simulink model "M10B39_V2"  (R2025a)
settings: Solver=ode23tb  StartTime=0.0  StopTime=1000  FixedStep=0.001  RelTol=1e-3  EnableMultiTasking=on
InitFcn:
  | clear;
  | initAll_V2;
  | %set_param('M10B39/Python2Sim','value','zeros(1,16)');
values from neighbouring files (symbols this model uses):
  acom = 100    [initAll.m]    (also in initAll_V2.m)
  bcom = 50    [initAll.m]    (also in initAll_V2.m)
  commun = 0*commun    [initAll.m]    (also in initAll_V2.m)
  DataDelay = 0.0*DataDelay    [initAll.m]    (also in initAll_V2.m)
  fB = 50    [initAll.m]    (also in initAll_V2.m)
  Geninit = Generator_init(opdata,SynMach_in_gidx)    [initAll.m]    (also in initAll_V2.m)
  lam = 100    [initAll.m]    (also in initAll_V2.m)
  loadnode = 31    [initAll_V2.m]
  loadsize = 16.2714    [initAll_V2.m]
  SgridB = 100    [initAll.m]    (also in initAll_V2.m)
  wB = 2*pi*fB    (= 314.159265359)    [initAll.m]    (also in initAll_V2.m)
undefined symbols (not defined in the file or in its folder): AVm0, c1, c2, c3, c4, c5, c6, cp_nom, ESinit, lambda_nom, P_wind_base, Pelec_base, Pnom, Windinit, YY_load
libraries: spsBistableLib x13, simulink_extras x5, powerlib_meascontrol x2, simulink x1
(part 3 of 11)

== system M10B39_V2/Network1 ==
  Ixy : Inport
  Assertion : Assertion  AssertionFailFcn=set_param(bdroot, 'SimulationCommand', 'pause')  StopWhenAssertionFail=off
  Clock : Clock
  Clock1 : Clock
  Constant : Constant  Value=0.001
  Mux : Mux  Inputs=2
  Relational Operator : RelationalOperator  Operator=<=  OutDataTypeStr=boolean  RndMeth=Simplest  InputSameDT=off
  Relational Operator1 : RelationalOperator  Operator=<=  OutDataTypeStr=boolean  RndMeth=Simplest  InputSameDT=off
  S-Function : S-Function  FunctionName=TS_net_1_new  Parameters=YY_load,ng,loadnode,loadsize  SFunctionDeploymentMode=off  EnableBusSupport=off
  S-Function Examples : simulink/User-Defined Functions/S-Function Examples  Commented=on
  S-Function1 : S-Function  Commented=on  Parameters=YY_load,ng  SFunctionDeploymentMode=off  EnableBusSupport=off
  Scope : Scope
      settings: ActiveDisplayYMinimum=0.9  ActiveDisplayYMaximum=1.1
  Sum : Sum  Inputs=|++
  pause_time : Constant  Value=1000
  Vxy : Outport
  wires:
  Ixy/1 -> Mux/2
  Mux/1 -> S-Function/1
  S-Function/1 -> Vxy/1
  Clock/1 -> Relational Operator/1, Mux/1
  Relational Operator/1 -> Assertion/1
  Clock1/1 -> Relational Operator1/1
  pause_time/1 -> Sum/1, Relational Operator/2
  Sum/1 -> Relational Operator1/2
  Relational Operator1/1 -> Scope/1
  Constant/1 -> Sum/2

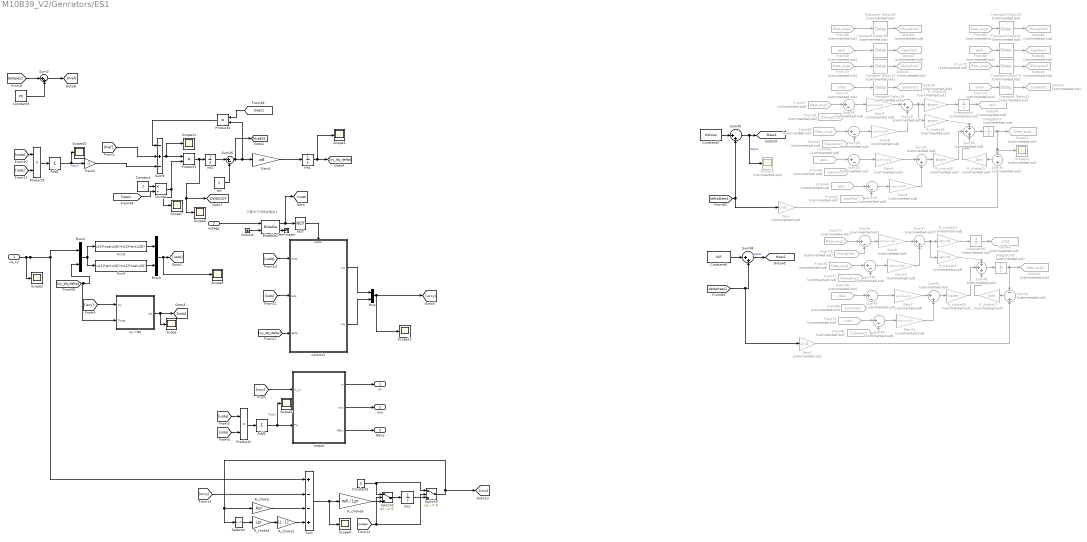
== system M10B39_V2/Genrators/ES1 ==
  note: 只要大于0就会输出1
  us_xy : Inport
  outage : Inport  Port=2
  " control1" : Subsystem
  Add1 : Sum  Inputs=+
  Add2 : Sum  Inputs=+
  Bistable2 : spsBistableLib/Bistable  Qpriority=Set  ic=0  Ts=0
      settings: LibrarySourceBlock=sps_lib/Control/Bistable
  Constant : Constant
  Constant1 : Constant  Value=0
  Constant3 : Constant  Value=P0
  Constant5 : Constant  Value=Kdroop
  Constant6 : Constant  Value=KIR
  Divide : Product  Inputs=*/
  Fcn3 : Fcn  Expr=u(1)*cos(u(3))+u(2)*sin(u(3))
  Fcn4 : Fcn  Expr=-u(1)*sin(u(3))+u(2)*cos(u(3))
  From57 : From  Commented=on  GotoTag=Dess_avg1  TagVisibility=global
  From58 : From  Commented=on  GotoTag=Dess_avg2  TagVisibility=global
  From59 : From  Commented=on  GotoTag=Dess_avg1  TagVisibility=global
  From60 : From  Commented=on  GotoTag=Dess_avg4  TagVisibility=global
  From61 : From  Commented=on  GotoTag=Davg2rec
  From62 : From  Commented=on  GotoTag=Davg4rec
  From63 : From  Commented=on  GotoTag=epi1  TagVisibility=global
  From64 : From  Commented=on  GotoTag=epi1  TagVisibility=global
  From66 : From  Commented=on  GotoTag=epi2rec
  From67 : From  Commented=on  GotoTag=epi4rec
  From68 : From  Commented=on  GotoTag=epi2  TagVisibility=global
  From69 : From  Commented=on  GotoTag=epi4  TagVisibility=global
  From70 : From  Commented=on  GotoTag=Hess_avg2  TagVisibility=global
  From71 : From  Commented=on  GotoTag=yita2  TagVisibility=global
  From72 : From  Commented=on  GotoTag=Hess_avg4  TagVisibility=global
  From73 : From  Commented=on  GotoTag=yita4  TagVisibility=global
  From74 : From  Commented=on  GotoTag=Hess_avg1  TagVisibility=global
  From75 : From  Commented=on  GotoTag=Hess_avg1  TagVisibility=global
  From76 : From  Commented=on  GotoTag=Havg2rec
  From77 : From  Commented=on  GotoTag=Havg4rec
  From78 : From  Commented=on  GotoTag=yita1  TagVisibility=global
  From79 : From  Commented=on  GotoTag=yita1  TagVisibility=global
  From80 : From  Commented=on  GotoTag=yita2rec
  From81 : From  Commented=on  GotoTag=yita4rec
  Gain : Gain  Commented=on  Gain=0.01
  Gain1 : Gain  Gain=wB  SaturateOnIntegerOverflow=on  OutDataTypeStr=Inherit: Same as input  ParamDataTypeStr=Inherit: Same as input
  Gain{8..11} (4 alike) : Gain  Commented=on  Gain=commun(4)
  Gain2 : Gain  Commented=on  Gain=0.01
  Gain{3,5..7} (4 alike) : Gain  Commented=on  Gain=commun(1)
  Gain4 : Gain  Gain=-1
  Goto32 : Goto  Commented=on  GotoTag=Dess_avg1  TagVisibility=global
  Goto33 : Goto  Commented=on  GotoTag=Havg2rec
  Goto34 : Goto  Commented=on  GotoTag=epi1  TagVisibility=global
  Goto35 : Goto  Commented=on  GotoTag=Davg2rec
  Goto36 : Goto  Commented=on  GotoTag=Davg4rec
  Goto37 : Goto  Commented=on  GotoTag=epi2rec
  Goto38 : Goto  Commented=on  GotoTag=epi4rec
  Goto39 : Goto  Commented=on  GotoTag=yita2rec
  Goto40 : Goto  Commented=on  GotoTag=Havg4rec
  Goto41 : Goto  Commented=on  GotoTag=yita4rec
  Goto42 : Goto  Commented=on  GotoTag=Hess_avg1  TagVisibility=global
  Goto43 : Goto  Commented=on  GotoTag=yita1  TagVisibility=global
  Ground : Ground
  Int1 : Integrator  InitialCondition=Dels_hvdc
  Int2 : Integrator  InitialCondition=1
  Integrator{6..9} (4 alike) : Integrator  Commented=on
  Isxy : Integrator  InitialCondition=[Is_xA_0 Is_yA_0]
  Mux : Mux  Inputs=2
  Mux3 : Mux  Inputs=2
  Mux4 : Mux  Inputs=2
  NOT : Logic  Operator=NOT  AllPortsSameDT=off  OutDataTypeStr=boolean
  Product1 : Product
  Product2 : Product  RndMeth=Zero
  Product3 : Product  RndMeth=Zero
  Product4 : Product
  R_choke : Gain  Gain=Rpr  SaturateOnIntegerOverflow=on  OutDataTypeStr=Inherit: Same as input  ParamDataTypeStr=Inherit: Same as input
  R_choke1 : Gain  Gain=Lpr  SaturateOnIntegerOverflow=on  OutDataTypeStr=Inherit: Same as input  ParamDataTypeStr=Inherit: Same as input
  R_choke14 : Gain  Commented=on  Gain=-bcom  SaturateOnIntegerOverflow=on  OutDataTypeStr=Inherit: Same as input  ParamDataTypeStr=Inherit: Same as input
  R_choke15 : Gain  Commented=on  Gain=-acom  SaturateOnIntegerOverflow=on  OutDataTypeStr=Inherit: Same as input  ParamDataTypeStr=Inherit: Same as input
  R_choke16 : Gain  Commented=on  Gain=bcom  SaturateOnIntegerOverflow=on  OutDataTypeStr=Inherit: Same as input  ParamDataTypeStr=Inherit: Same as input
  R_choke17 : Gain  Commented=on  Gain=lam  SaturateOnIntegerOverflow=on  OutDataTypeStr=Inherit: Same as input  ParamDataTypeStr=Inherit: Same as input
  R_choke18 : Gain  Commented=on  Gain=-bcom  SaturateOnIntegerOverflow=on  OutDataTypeStr=Inherit: Same as input  ParamDataTypeStr=Inherit: Same as input
  R_choke19 : Gain  Commented=on  Gain=-acom  SaturateOnIntegerOverflow=on  OutDataTypeStr=Inherit: Same as input  ParamDataTypeStr=Inherit: Same as input
  R_choke2 : Gain  Gain=[1 -1]  SaturateOnIntegerOverflow=on  OutDataTypeStr=Inherit: Same as input  ParamDataTypeStr=Inherit: Same as input
  R_choke20 : Gain  Commented=on  Gain=bcom  SaturateOnIntegerOverflow=on  OutDataTypeStr=Inherit: Same as input  ParamDataTypeStr=Inherit: Same as input
  R_choke21 : Gain  Commented=on  Gain=lam  SaturateOnIntegerOverflow=on  OutDataTypeStr=Inherit: Same as input  ParamDataTypeStr=Inherit: Same as input
  R_choke3 : Gain  Gain=wB / Lpr  SaturateOnIntegerOverflow=on  OutDataTypeStr=Inherit: Same as input  ParamDataTypeStr=Inherit: Same as input
  Scope{,1..7,10..12} (11 alike) : Scope
      Scope settings: ActiveDisplayYMinimum=-0.0194  ActiveDisplayYMaximum=0.04689
      Scope1 settings: DataLoggingVariableName=ScopeData16
      Scope10 settings: ActiveDisplayYMinimum=-5.21032  ActiveDisplayYMaximum=-1.08346
      Scope11 settings: ActiveDisplayYMinimum=-0.1125  ActiveDisplayYMaximum=0.0125  DataLoggingVariableName=ScopeData2
      Scope12 settings: ActiveDisplayYMinimum=0.46883  ActiveDisplayYMaximum=1.25548  DataLoggingVariableName=ScopeData3
      Scope2 settings: DataLoggingVariableName=ScopeData17
      Scope3 settings: ActiveDisplayYMinimum=-0.44976  ActiveDisplayYMaximum=2.17603
      Scope4 settings: ActiveDisplayYMinimum=-2.8E-5  ActiveDisplayYMaximum=2.4E-5  DataLoggingVariableName=ScopeData5
      Scope5 settings: ActiveDisplayYMinimum=-2.50000000003  ActiveDisplayYMaximum=-2.49999999989  DataLoggingVariableName=ScopeData7
      Scope6 settings: ActiveDisplayYMinimum=-0.00021  ActiveDisplayYMaximum=0.0004  DataLoggingVariableName=ScopeData4
      Scope7 settings: ActiveDisplayYMinimum=0.9  ActiveDisplayYMaximum=1.1  DataLoggingVariableName=ScopeData14
  Scope14 : Scope  Commented=on
      settings: ActiveDisplayYMinimum=-0.0418  ActiveDisplayYMaximum=0.37621  DataLoggingVariableName=ScopeData2
  Scope15 : Scope  Commented=on
      settings: ActiveDisplayYMinimum=-1  ActiveDisplayYMaximum=1  DataLoggingVariableName=ScopeData3
  Selector : Selector  InputPortWidth=2  IndexOptions=Index vector (dialog)  Indices=[2 1]  OutputSizes=1
  Sum : Sum  Inputs=+--+  SaturateOnIntegerOverflow=on
  Sum2 : Sum  Inputs=|++
  Sum26 : Sum  Inputs=|+-  SaturateOnIntegerOverflow=on
  Sum{28,30,32,34,36,39,41,43} (8 alike) : Sum  Commented=on  Inputs=|+-  SaturateOnIntegerOverflow=on
  Sum{29,33,37,42} (4 alike) : Sum  Commented=on  Inputs=|++  SaturateOnIntegerOverflow=on
  Sum31 : Sum  Commented=on  Inputs=+++  SaturateOnIntegerOverflow=on
  Sum35 : Sum  Commented=on  Inputs=-+  SaturateOnIntegerOverflow=on
  Sum38 : Sum  Inputs=|++  SaturateOnIntegerOverflow=on
  Sum40 : Sum  Commented=on  Inputs=+++  SaturateOnIntegerOverflow=on
  Sum44 : Sum  Commented=on  Inputs=-+  SaturateOnIntegerOverflow=on
  Sum45 : Sum  Inputs=|++  SaturateOnIntegerOverflow=on
  Sum9 : Sum  Inputs=-+-  SaturateOnIntegerOverflow=on
  Switch2 : Switch  Criteria=u2 ~= 0  Threshold=0.5  InputSameDT=off
  Switch3 : Switch  Criteria=u2 ~= 0  Threshold=0.5  InputSameDT=off
  Terminator : Terminator
  Transport Delay{14..15,19,21} (4 alike) : TransportDelay  Commented=on  DelayTime=DataDelay(4,2)
  Transport Delay{18,20,22..23} (4 alike) : TransportDelay  Commented=on  DelayTime=DataDelay(2,1)
  output : Subsystem
  w0 : Constant
  xy->dq : Subsystem
  m : Outport
  isxy : Outport  Port=2
  GBxy : Outport  Port=3
  tag scope: DWES1DT=global, Dess1=global, Hess1=global, WreES1=global
  wires:
  Selector/1 -> R_choke1/1
  Sum/1 -> Scope4/1, R_choke3/1
  R_choke3/1 -> Switch2/3
  Ground/1 -> Bistable2/2
  R_choke2/1 -> Sum/4
  R_choke/1 -> Sum/3
  [ucxy] -> Sum/2
  output/1(m) -> m/1
  NOT/1 -> " control1"/Enable
  R_choke1/1 -> R_choke2/1
  Bistable2/1 -> NOT/1, [outage]
  Isxy/1 -> Switch3/3
  [isxy] -> xy->dq/1(Ixy)
  [isxy] -> output/1(is_xy)
  output/2(isxy) -> isxy/1
  [xy_dq_delta] -> " control1"/3(delta)
  xy->dq/1(Idq) -> [isdq], Scope/1
  Bistable2/2 -> Terminator/1
  outage/1 -> Bistable2/1
  [outage] -> Switch2/2, Switch3/2
  [isdq] -> " control1"/2(isdq)
  " control1"/1(ucx) -> Mux/1
  Switch2/1 -> Isxy/1
  Switch3/1 -> R_choke/1, Selector/1, [isxy]
  Mux/1 -> Scope12/1, [ucxy]
  [usdq] -> " control1"/1(usdq)
  output/3(GBxy) -> GBxy/1
  Constant1/1 -> Switch2/1, Switch3/1
  " control1"/2(ucy) -> Mux/2
  [usdq] -> Product2/1
  Add1/1 -> Scope5/1, output/2(Pe)  "Pess1"
  Product2/1 -> Add1/1
  [isdq] -> Product2/2
  Product1/1 -> Scope6/1, [DWES1DT], Int2/1
  Sum26/1 -> [WreES1], Product4/2, Gain1/1
  Int2/1 -> Sum26/1
  w0/1 -> Sum26/2
  Sum9/1 -> Product1/1, Scope11/1
  Constant/1 -> Divide/1
  Divide/1 -> Product1/2, Scope7/1
  [Hess1] -> Divide/2
  us_xy/1 -> Scope2/1, Mux4/1, Sum/1
  Fcn3/1 -> Mux3/1
  Fcn4/1 -> Mux3/2
  Mux4/1 -> Fcn3/1, Fcn4/1
  [xy_dq_delta] -> Mux4/2, xy->dq/2(Theta)
  Mux3/1 -> Scope3/1, [usdq]
  Gain4/1 -> Sum9/3
  Product4/1 -> Sum9/1
  Int1/1 -> Scope1/1, [xy_dq_delta]
  Add2/1 -> Gain4/1, Scope10/1  "Pess1"
  [usdq] -> Product3/1
  [isdq] -> Product3/2
  Product3/1 -> Add2/1
  Transport Delay19/1 -> Goto36/1
  R_choke20/1 -> Sum31/2
  R_choke19/1 -> Sum31/1
  From57/1 -> Sum28/1
  From59/1 -> Sum30/1
  Sum38/1 -> [Hess1]  "Hess1"
  Sum45/1 -> Scope15/1, [Dess1]  "Dess1"
  Constant6/1 -> Sum38/1
  From64/1 -> Sum34/1
  R_choke21/1 -> Sum31/3
  Integrator6/1 -> Goto34/1
  Sum35/1 -> R_choke21/1
  Sum31/1 -> Integrator7/1
  Integrator7/1 -> Goto32/1, Scope14/1, Sum35/1
  Transport Delay21/1 -> Goto38/1
  From68/1 -> Transport Delay20/1
  From67/1 -> Sum34/2
  From62/1 -> Sum30/2
  From80/1 -> Sum41/2
  From78/1 -> Sum41/1
  Sum40/1 -> Integrator9/1
  [deltaDess1] -> Sum45/2, Gain/1
  R_choke18/1 -> Integrator6/1
  From77/1 -> Sum39/2
  From63/1 -> Sum32/1
  From76/1 -> Sum36/2
  Sum42/1 -> R_choke16/1
  From58/1 -> Transport Delay18/1
  Transport Delay20/1 -> Goto37/1
  Transport Delay14/1 -> Goto40/1
  From75/1 -> Sum39/1
  Integrator9/1 -> Goto42/1, Sum44/1
  Sum29/1 -> R_choke19/1, R_choke18/1
  From61/1 -> Sum28/2
  From71/1 -> Transport Delay23/1
  Sum37/1 -> R_choke15/1, R_choke14/1
  R_choke14/1 -> Integrator8/1
  Integrator8/1 -> Goto43/1
  Transport Delay18/1 -> Goto35/1
  R_choke17/1 -> Sum40/3
  R_choke15/1 -> Sum40/1
  R_choke16/1 -> Sum40/2
  From74/1 -> Sum36/1
  [deltaHess1] -> Sum38/2, Gain2/1
  Sum44/1 -> R_choke17/1
  Sum33/1 -> R_choke20/1
  Transport Delay23/1 -> Goto39/1
  From66/1 -> Sum32/2
  Transport Delay22/1 -> Goto33/1
  Transport Delay15/1 -> Goto41/1
  From70/1 -> Transport Delay22/1
  [Dess1] -> Product4/1
  Gain1/1 -> Int1/1
  From81/1 -> Sum43/2
  From79/1 -> Sum43/1
  Gain/1 -> Sum35/2
  Gain2/1 -> Sum44/2
  From60/1 -> Transport Delay19/1
  From69/1 -> Transport Delay21/1
  From72/1 -> Transport Delay14/1
  From73/1 -> Transport Delay15/1
  Gain3/1 -> Sum29/1
  Sum28/1 -> Gain3/1
  Gain5/1 -> Sum33/1
  Sum32/1 -> Gain5/1
  Sum36/1 -> Gain6/1
  Gain6/1 -> Sum37/1
  Gain7/1 -> Sum42/1
  Sum41/1 -> Gain7/1
  Sum30/1 -> Gain8/1
  Gain8/1 -> Sum29/2
  Sum34/1 -> Gain9/1
  Gain9/1 -> Sum33/2
  Sum39/1 -> Gain10/1
  Gain10/1 -> Sum37/2
  Sum43/1 -> Gain11/1
  Gain11/1 -> Sum42/2
  Constant5/1 -> Sum45/1
  [deltapes1] -> Sum2/1
  Constant3/1 -> Sum2/2
  Sum2/1 -> [Pref]
  [Pref] -> Sum9/2

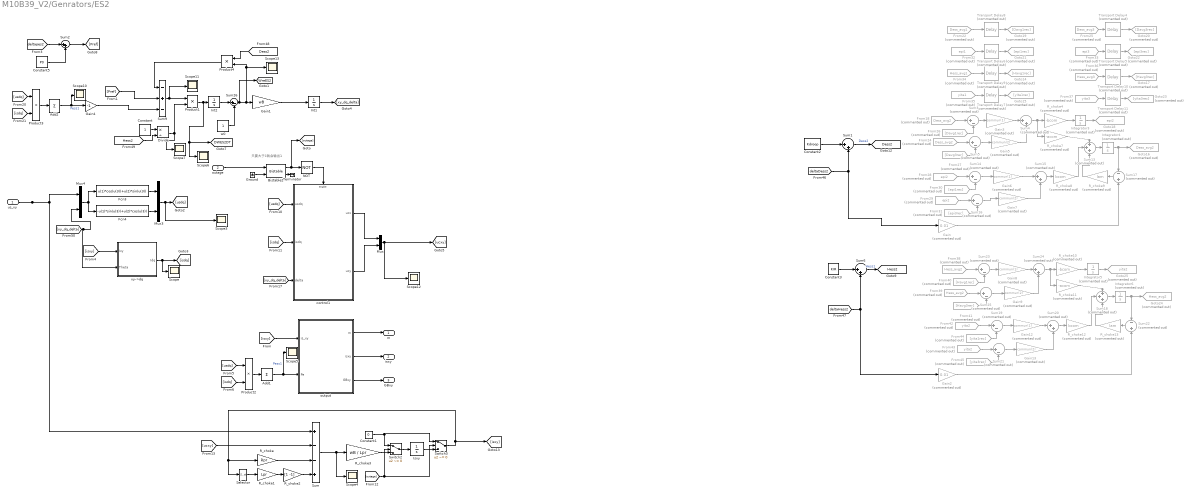
== system M10B39_V2/Genrators/ES2 ==
  note: 只要大于0就会输出1
  us_xy : Inport
  outage : Inport  Port=2
  " control1" : Subsystem
  Add1 : Sum  Inputs=+
  Add2 : Sum  Inputs=+
  Bistable2 : spsBistableLib/Bistable  Qpriority=Set  ic=0  Ts=0
      settings: LibrarySourceBlock=sps_lib/Control/Bistable
  Constant : Constant
  Constant1 : Constant  Value=0
  Constant2 : Constant  Value=Kdroop
  Constant3 : Constant  Value=KIR
  Constant5 : Constant  Value=P0
  Divide : Product  Inputs=*/
  Fcn3 : Fcn  Expr=u(1)*cos(u(3))+u(2)*sin(u(3))
  Fcn4 : Fcn  Expr=-u(1)*sin(u(3))+u(2)*cos(u(3))
  From18 : From  Commented=on  GotoTag=Dess_avg2  TagVisibility=global
  From22 : From  Commented=on  GotoTag=Dess_avg1  TagVisibility=global
  From24 : From  Commented=on  GotoTag=Dess_avg2  TagVisibility=global
  From25 : From  Commented=on  GotoTag=Dess_avg3  TagVisibility=global
  From26 : From  Commented=on  GotoTag=Davg1rec
  From27 : From  Commented=on  GotoTag=Davg3rec
  From28 : From  Commented=on  GotoTag=epi2  TagVisibility=global
  From29 : From  Commented=on  GotoTag=epi2  TagVisibility=global
  From30 : From  Commented=on  GotoTag=epi1rec
  From31 : From  Commented=on  GotoTag=epi3rec
  From32 : From  Commented=on  GotoTag=epi1  TagVisibility=global
  From33 : From  Commented=on  GotoTag=epi3  TagVisibility=global
  From34 : From  Commented=on  GotoTag=Hess_avg1  TagVisibility=global
  From35 : From  Commented=on  GotoTag=yita1  TagVisibility=global
  From36 : From  Commented=on  GotoTag=Hess_avg3  TagVisibility=global
  From37 : From  Commented=on  GotoTag=yita3  TagVisibility=global
  From38 : From  Commented=on  GotoTag=Hess_avg2  TagVisibility=global
  From39 : From  Commented=on  GotoTag=Hess_avg2  TagVisibility=global
  From40 : From  Commented=on  GotoTag=Havg1rec
  From41 : From  Commented=on  GotoTag=Havg3rec
  From42 : From  Commented=on  GotoTag=yita2  TagVisibility=global
  From43 : From  Commented=on  GotoTag=yita2  TagVisibility=global
  From44 : From  Commented=on  GotoTag=yita1rec
  From45 : From  Commented=on  GotoTag=yita3rec
  Gain : Gain  Commented=on  Gain=0.01
  Gain1 : Gain  Gain=wB  SaturateOnIntegerOverflow=on  OutDataTypeStr=Inherit: Same as input  ParamDataTypeStr=Inherit: Same as input
  Gain{3,6,8,12} (4 alike) : Gain  Commented=on  Gain=commun(1)
  Gain{5,7,9,13} (4 alike) : Gain  Commented=on  Gain=commun(2)
  Gain2 : Gain  Commented=on  Gain=0.01
  Gain4 : Gain  Gain=-1
  Goto14 : Goto  Commented=on  GotoTag=Havg1rec
  Goto15 : Goto  Commented=on  GotoTag=yita1rec
  Goto16 : Goto  Commented=on  GotoTag=Dess_avg2  TagVisibility=global
  Goto17 : Goto  Commented=on  GotoTag=Havg3rec
  Goto18 : Goto  Commented=on  GotoTag=epi2  TagVisibility=global
  Goto19 : Goto  Commented=on  GotoTag=Davg1rec
  Goto20 : Goto  Commented=on  GotoTag=Davg3rec
  Goto21 : Goto  Commented=on  GotoTag=epi1rec
  Goto22 : Goto  Commented=on  GotoTag=epi3rec
  Goto23 : Goto  Commented=on  GotoTag=yita3rec
  Goto24 : Goto  Commented=on  GotoTag=Hess_avg2  TagVisibility=global
  Goto25 : Goto  Commented=on  GotoTag=yita2  TagVisibility=global
  Ground : Ground
  Int1 : Integrator  InitialCondition=Dels_hvdc
  Int2 : Integrator  InitialCondition=1
  Integrator{3..6} (4 alike) : Integrator  Commented=on
  Isxy : Integrator  InitialCondition=[Is_xA_0 Is_yA_0]
  Mux : Mux  Inputs=2
  Mux3 : Mux  Inputs=2
  Mux4 : Mux  Inputs=2
  NOT : Logic  Operator=NOT  AllPortsSameDT=off  OutDataTypeStr=boolean
  Product1 : Product
  Product2 : Product  RndMeth=Zero
  Product3 : Product  RndMeth=Zero
  Product4 : Product
  R_choke : Gain  Gain=Rpr  SaturateOnIntegerOverflow=on  OutDataTypeStr=Inherit: Same as input  ParamDataTypeStr=Inherit: Same as input
  R_choke1 : Gain  Gain=Lpr  SaturateOnIntegerOverflow=on  OutDataTypeStr=Inherit: Same as input  ParamDataTypeStr=Inherit: Same as input
  R_choke10 : Gain  Commented=on  Gain=-bcom  SaturateOnIntegerOverflow=on  OutDataTypeStr=Inherit: Same as input  ParamDataTypeStr=Inherit: Same as input
  R_choke11 : Gain  Commented=on  Gain=-acom  SaturateOnIntegerOverflow=on  OutDataTypeStr=Inherit: Same as input  ParamDataTypeStr=Inherit: Same as input
  R_choke12 : Gain  Commented=on  Gain=bcom  SaturateOnIntegerOverflow=on  OutDataTypeStr=Inherit: Same as input  ParamDataTypeStr=Inherit: Same as input
  R_choke13 : Gain  Commented=on  Gain=lam  SaturateOnIntegerOverflow=on  OutDataTypeStr=Inherit: Same as input  ParamDataTypeStr=Inherit: Same as input
  R_choke2 : Gain  Gain=[1 -1]  SaturateOnIntegerOverflow=on  OutDataTypeStr=Inherit: Same as input  ParamDataTypeStr=Inherit: Same as input
  R_choke3 : Gain  Gain=wB / Lpr  SaturateOnIntegerOverflow=on  OutDataTypeStr=Inherit: Same as input  ParamDataTypeStr=Inherit: Same as input
  R_choke4 : Gain  Commented=on  Gain=-bcom  SaturateOnIntegerOverflow=on  OutDataTypeStr=Inherit: Same as input  ParamDataTypeStr=Inherit: Same as input
  R_choke7 : Gain  Commented=on  Gain=-acom  SaturateOnIntegerOverflow=on  OutDataTypeStr=Inherit: Same as input  ParamDataTypeStr=Inherit: Same as input
  R_choke8 : Gain  Commented=on  Gain=bcom  SaturateOnIntegerOverflow=on  OutDataTypeStr=Inherit: Same as input  ParamDataTypeStr=Inherit: Same as input
  R_choke9 : Gain  Commented=on  Gain=lam  SaturateOnIntegerOverflow=on  OutDataTypeStr=Inherit: Same as input  ParamDataTypeStr=Inherit: Same as input
  Scope{,3..7,10..13} (10 alike) : Scope
      Scope settings: ActiveDisplayYMinimum=-0.0194  ActiveDisplayYMaximum=0.04689
      Scope10 settings: ActiveDisplayYMinimum=-0.00511  ActiveDisplayYMaximum=0.046
      Scope11 settings: ActiveDisplayYMinimum=-0.1125  ActiveDisplayYMaximum=0.0125  DataLoggingVariableName=ScopeData2
      Scope12 settings: ActiveDisplayYMinimum=0.46883  ActiveDisplayYMaximum=1.25548  DataLoggingVariableName=ScopeData3
      Scope13 settings: ActiveDisplayYMinimum=-0.0063  ActiveDisplayYMaximum=0.05669  DataLoggingVariableName=ScopeData4
      Scope3 settings: ActiveDisplayYMinimum=-0.12696  ActiveDisplayYMaximum=1.14248
      Scope4 settings: ActiveDisplayYMinimum=-2.8E-5  ActiveDisplayYMaximum=2.4E-5  DataLoggingVariableName=ScopeData5
      Scope5 settings: ActiveDisplayYMinimum=-0.00823  ActiveDisplayYMaximum=0.07404  DataLoggingVariableName=ScopeData7
      Scope6 settings: ActiveDisplayYMinimum=-0.00105  ActiveDisplayYMaximum=0.00091  DataLoggingVariableName=ScopeData4
      Scope7 settings: ActiveDisplayYMinimum=0.9  ActiveDisplayYMaximum=1.1  DataLoggingVariableName=ScopeData14
  Selector : Selector  InputPortWidth=2  IndexOptions=Index vector (dialog)  Indices=[2 1]  OutputSizes=1
  Sum : Sum  Inputs=+--+  SaturateOnIntegerOverflow=on
  Sum1 : Sum  Inputs=|++  SaturateOnIntegerOverflow=on
  Sum13 : Sum  Commented=on  Inputs=+++  SaturateOnIntegerOverflow=on
  Sum{3,5,14,16,19,21,23,25} (8 alike) : Sum  Commented=on  Inputs=|+-  SaturateOnIntegerOverflow=on
  Sum{4,15,20,24} (4 alike) : Sum  Commented=on  Inputs=|++  SaturateOnIntegerOverflow=on
  Sum17 : Sum  Commented=on  Inputs=-+  SaturateOnIntegerOverflow=on
  Sum18 : Sum  Commented=on  Inputs=+++  SaturateOnIntegerOverflow=on
  Sum2 : Sum  Inputs=|++
  Sum22 : Sum  Commented=on  Inputs=-+  SaturateOnIntegerOverflow=on
  Sum26 : Sum  Inputs=|+-  SaturateOnIntegerOverflow=on
  Sum6 : Sum  Inputs=|++  SaturateOnIntegerOverflow=on
  Sum9 : Sum  Inputs=-+-  SaturateOnIntegerOverflow=on
  Switch2 : Switch  Criteria=u2 ~= 0  Threshold=0.5  InputSameDT=off
  Switch3 : Switch  Criteria=u2 ~= 0  Threshold=0.5  InputSameDT=off
  Terminator : Terminator
  Transport Delay{4..5,10..11} (4 alike) : TransportDelay  Commented=on  DelayTime=DataDelay(3,1)
  Transport Delay{6..9} (4 alike) : TransportDelay  Commented=on  DelayTime=DataDelay(1,2)
  output : Subsystem
  w0 : Constant
  xy->dq : Subsystem
  m : Outport
  isxy : Outport  Port=2
  GBxy : Outport  Port=3
  tag scope: DWES2DT=global, Dess2=global, Hess2=global, WreES2=global
  wires:
  Selector/1 -> R_choke1/1
  Sum/1 -> Scope4/1, R_choke3/1
  R_choke3/1 -> Switch2/3
  Ground/1 -> Bistable2/2
  R_choke2/1 -> Sum/4
  R_choke/1 -> Sum/3
  [ucxy] -> Sum/2
  output/1(m) -> m/1
  NOT/1 -> " control1"/Enable
  R_choke1/1 -> R_choke2/1
  Bistable2/1 -> NOT/1, [outage]
  Isxy/1 -> Switch3/3
  [isxy] -> xy->dq/1(Ixy)
  [isxy] -> output/1(is_xy)
  output/2(isxy) -> isxy/1
  [xy_dq_delta] -> " control1"/3(delta)
  xy->dq/1(Idq) -> [isdq], Scope/1
  Bistable2/2 -> Terminator/1
  outage/1 -> Bistable2/1
  [outage] -> Switch2/2, Switch3/2
  [isdq] -> " control1"/2(isdq)
  " control1"/1(ucx) -> Mux/1
  Switch2/1 -> Isxy/1
  Switch3/1 -> R_choke/1, Selector/1, [isxy]
  Mux/1 -> Scope12/1, [ucxy]
  [usdq] -> " control1"/1(usdq)
  output/3(GBxy) -> GBxy/1
  Constant1/1 -> Switch2/1, Switch3/1
  " control1"/2(ucy) -> Mux/2
  [usdq] -> Product2/1
  Add1/1 -> output/2(Pe), Scope5/1  "Pess1"
  Product2/1 -> Add1/1
  [isdq] -> Product2/2
  Product1/1 -> Scope6/1, [DWES2DT], Int2/1
  Sum26/1 -> [WreES2], Scope13/1, Product4/2, Gain1/1
  Int2/1 -> Sum26/1
  w0/1 -> Sum26/2
  Sum9/1 -> Product1/1, Scope11/1
  Constant/1 -> Divide/1
  Divide/1 -> Product1/2, Scope7/1
  [Hess2] -> Divide/2
  us_xy/1 -> Mux4/1, Sum/1
  Fcn3/1 -> Mux3/1
  Fcn4/1 -> Mux3/2
  Mux4/1 -> Fcn3/1, Fcn4/1
  [xy_dq_delta] -> Mux4/2, xy->dq/2(Theta)
  Mux3/1 -> Scope3/1, [usdq]
  Gain4/1 -> Sum9/3
  [Pref] -> Sum9/2
  Product4/1 -> Sum9/1
  Int1/1 -> [xy_dq_delta]
  Add2/1 -> Gain4/1, Scope10/1  "Pess1"
  [usdq] -> Product3/1
  [isdq] -> Product3/2
  Product3/1 -> Add2/1
  [Dess2] -> Product4/1
  Gain1/1 -> Int1/1
  From27/1 -> Sum5/2
  R_choke7/1 -> Sum13/1
  From44/1 -> Sum19/2
  R_choke8/1 -> Sum13/2
  From24/1 -> Sum5/1
  From18/1 -> Sum3/1
  Transport Delay9/1 -> Goto14/1
  From26/1 -> Sum3/2
  Transport Delay6/1 -> Goto21/1
  Integrator3/1 -> Goto18/1
  From30/1 -> Sum14/2
  Transport Delay5/1 -> Goto22/1
  Sum20/1 -> R_choke12/1
  Transport Delay4/1 -> Goto20/1
  From43/1 -> Sum21/1
  Transport Delay7/1 -> Goto15/1
  Sum17/1 -> R_choke9/1
  [deltaDess2] -> Sum1/2, Gain/1
  From39/1 -> Sum25/1
  Sum13/1 -> Integrator4/1
  R_choke10/1 -> Integrator5/1
  Sum15/1 -> R_choke8/1
  R_choke9/1 -> Sum13/3
  Constant3/1 -> Sum6/1
  Integrator4/1 -> Goto16/1, Sum17/1
  From29/1 -> Sum16/1
  [deltaHess2] -> Sum6/2, Gain2/1
  Transport Delay10/1 -> Goto17/1
  From31/1 -> Sum16/2
  Sum24/1 -> R_choke11/1, R_choke10/1
  Sum6/1 -> [Hess2]  "Hess1"
  From42/1 -> Sum19/1
  From28/1 -> Sum14/1
  R_choke12/1 -> Sum18/2
  From38/1 -> Sum23/1
  R_choke11/1 -> Sum18/1
  R_choke4/1 -> Integrator3/1
  Sum4/1 -> R_choke7/1, R_choke4/1
  From45/1 -> Sum21/2
  From40/1 -> Sum23/2
  From41/1 -> Sum25/2
  Transport Delay11/1 -> Goto23/1
  Sum22/1 -> R_choke13/1
  Integrator6/1 -> Goto24/1, Sum22/1
  Sum18/1 -> Integrator6/1
  Integrator5/1 -> Goto25/1
  R_choke13/1 -> Sum18/3
  Transport Delay8/1 -> Goto19/1
  Sum1/1 -> [Dess2]  "Dess2"
  Constant2/1 -> Sum1/1
  Gain/1 -> Sum17/2
  Gain2/1 -> Sum22/2
  From22/1 -> Transport Delay8/1
  From32/1 -> Transport Delay6/1
  From34/1 -> Transport Delay9/1
  From35/1 -> Transport Delay7/1
  From25/1 -> Transport Delay4/1
  From33/1 -> Transport Delay5/1
  From36/1 -> Transport Delay10/1
  From37/1 -> Transport Delay11/1
  Gain3/1 -> Sum4/1
  Sum3/1 -> Gain3/1
  Sum5/1 -> Gain5/1
  Gain5/1 -> Sum4/2
  Gain6/1 -> Sum15/1
  Sum14/1 -> Gain6/1
  Sum16/1 -> Gain7/1
  Gain7/1 -> Sum15/2
  Sum23/1 -> Gain8/1
  Gain8/1 -> Sum24/1
  Sum25/1 -> Gain9/1
  Gain9/1 -> Sum24/2
  Gain12/1 -> Sum20/1
  Sum19/1 -> Gain12/1
  Sum21/1 -> Gain13/1
  Gain13/1 -> Sum20/2
  Constant5/1 -> Sum2/2
  Sum2/1 -> [Pref]
  [deltapes2] -> Sum2/1

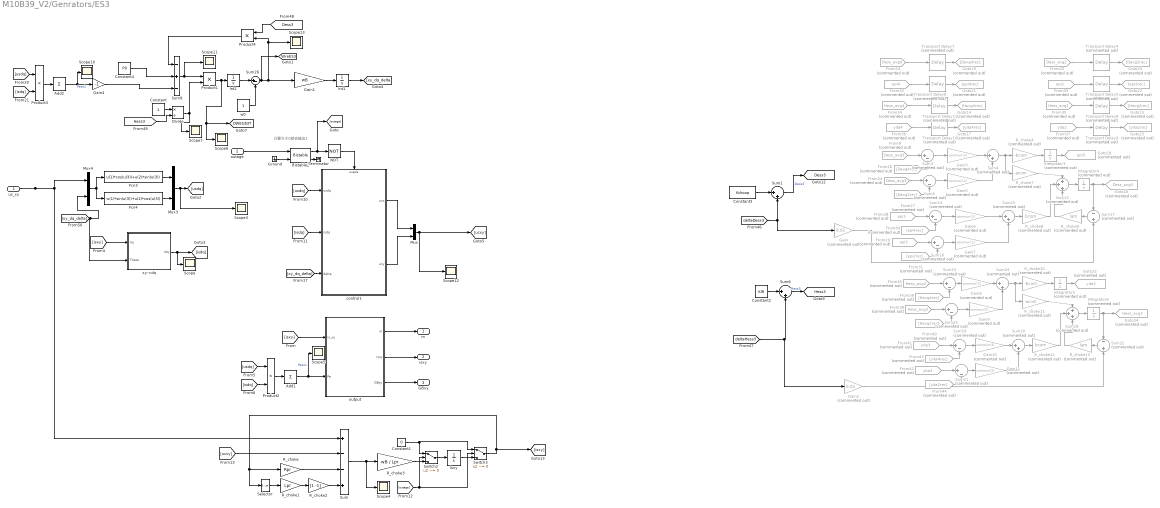
== system M10B39_V2/Genrators/ES3 ==
  note: 只要大于0就会输出1
  us_xy : Inport
  outage : Inport  Port=2
  " control1" : Subsystem
  Add1 : Sum  Inputs=+
  Add2 : Sum  Inputs=+
  Bistable2 : powerlib_meascontrol/Logic/Bistable  Qpriority=Set  ic=0  Ts=0
  Constant : Constant
  Constant1 : Constant  Value=0
  Constant2 : Constant  Value=KIR
  Constant3 : Constant  Value=Kdroop
  Constant4 : Constant  Value=P0
  Divide : Product  Inputs=*/
  Fcn3 : Fcn  Expr=u(1)*cos(u(3))+u(2)*sin(u(3))
  Fcn4 : Fcn  Expr=-u(1)*sin(u(3))+u(2)*cos(u(3))
  From14 : From  Commented=on  GotoTag=Dess_avg4  TagVisibility=global
  From24 : From  Commented=on  GotoTag=Dess_avg3  TagVisibility=global
  From25 : From  Commented=on  GotoTag=Dess_avg2  TagVisibility=global
  From26 : From  Commented=on  GotoTag=Davg4rec
  From27 : From  Commented=on  GotoTag=Davg2rec
  From28 : From  Commented=on  GotoTag=epi3  TagVisibility=global
  From29 : From  Commented=on  GotoTag=epi3  TagVisibility=global
  From30 : From  Commented=on  GotoTag=epi4rec
  From31 : From  Commented=on  GotoTag=epi2rec
  From32 : From  Commented=on  GotoTag=epi4  TagVisibility=global
  From33 : From  Commented=on  GotoTag=epi2  TagVisibility=global
  From34 : From  Commented=on  GotoTag=Hess_avg4  TagVisibility=global
  From35 : From  Commented=on  GotoTag=Hess_avg2  TagVisibility=global
  From36 : From  Commented=on  GotoTag=yita4  TagVisibility=global
  From37 : From  Commented=on  GotoTag=yita2  TagVisibility=global
  From38 : From  Commented=on  GotoTag=Hess_avg3  TagVisibility=global
  From39 : From  Commented=on  GotoTag=Havg4rec
  From40 : From  Commented=on  GotoTag=Havg2rec
  From41 : From  Commented=on  GotoTag=yita3  TagVisibility=global
  From42 : From  Commented=on  GotoTag=yita3  TagVisibility=global
  From43 : From  Commented=on  GotoTag=yita4rec
  From44 : From  Commented=on  GotoTag=yita2rec
  From45 : From  Commented=on  GotoTag=Hess_avg3  TagVisibility=global
  From9 : From  Commented=on  GotoTag=Dess_avg3  TagVisibility=global
  Gain : Gain  Commented=on  Gain=0.01
  Gain1 : Gain  Gain=wB  SaturateOnIntegerOverflow=on  OutDataTypeStr=Inherit: Same as input  ParamDataTypeStr=Inherit: Same as input
  Gain{3,6,8,10} (4 alike) : Gain  Commented=on  Gain=commun(3)
  Gain{5,7,9,11} (4 alike) : Gain  Commented=on  Gain=commun(2)
  Gain2 : Gain  Commented=on  Gain=0.01
  Gain4 : Gain  Gain=-1
  Goto14 : Goto  Commented=on  GotoTag=Havg4rec
  Goto15 : Goto  Commented=on  GotoTag=Havg2rec
  Goto16 : Goto  Commented=on  GotoTag=Dess_avg3  TagVisibility=global
  Goto17 : Goto  Commented=on  GotoTag=yita4rec
  Goto18 : Goto  Commented=on  GotoTag=epi3  TagVisibility=global
  Goto19 : Goto  Commented=on  GotoTag=Davg4rec
  Goto20 : Goto  Commented=on  GotoTag=Davg2rec
  Goto21 : Goto  Commented=on  GotoTag=epi4rec
  Goto22 : Goto  Commented=on  GotoTag=epi2rec
  Goto23 : Goto  Commented=on  GotoTag=yita2rec
  Goto24 : Goto  Commented=on  GotoTag=Hess_avg3  TagVisibility=global
  Goto25 : Goto  Commented=on  GotoTag=yita3  TagVisibility=global
  Ground : Ground
  Int1 : Integrator  InitialCondition=Dels_hvdc
  Int2 : Integrator  InitialCondition=1
  Integrator{3..6} (4 alike) : Integrator  Commented=on
  Isxy : Integrator  InitialCondition=[Is_xA_0 Is_yA_0]
  Mux : Mux  Inputs=2
  Mux3 : Mux  Inputs=2
  Mux4 : Mux  Inputs=2
  NOT : Logic  Operator=NOT  AllPortsSameDT=off  OutDataTypeStr=boolean
  Product1 : Product
  Product2 : Product  RndMeth=Zero
  Product3 : Product  RndMeth=Zero
  Product4 : Product
  R_choke : Gain  Gain=Rpr  SaturateOnIntegerOverflow=on  OutDataTypeStr=Inherit: Same as input  ParamDataTypeStr=Inherit: Same as input
  R_choke1 : Gain  Gain=Lpr  SaturateOnIntegerOverflow=on  OutDataTypeStr=Inherit: Same as input  ParamDataTypeStr=Inherit: Same as input
  R_choke10 : Gain  Commented=on  Gain=-bcom  SaturateOnIntegerOverflow=on  OutDataTypeStr=Inherit: Same as input  ParamDataTypeStr=Inherit: Same as input
  R_choke11 : Gain  Commented=on  Gain=-acom  SaturateOnIntegerOverflow=on  OutDataTypeStr=Inherit: Same as input  ParamDataTypeStr=Inherit: Same as input
  R_choke12 : Gain  Commented=on  Gain=bcom  SaturateOnIntegerOverflow=on  OutDataTypeStr=Inherit: Same as input  ParamDataTypeStr=Inherit: Same as input
  R_choke13 : Gain  Commented=on  Gain=lam  SaturateOnIntegerOverflow=on  OutDataTypeStr=Inherit: Same as input  ParamDataTypeStr=Inherit: Same as input
  R_choke2 : Gain  Gain=[1 -1]  SaturateOnIntegerOverflow=on  OutDataTypeStr=Inherit: Same as input  ParamDataTypeStr=Inherit: Same as input
  R_choke3 : Gain  Gain=wB / Lpr  SaturateOnIntegerOverflow=on  OutDataTypeStr=Inherit: Same as input  ParamDataTypeStr=Inherit: Same as input
  R_choke4 : Gain  Commented=on  Gain=-bcom  SaturateOnIntegerOverflow=on  OutDataTypeStr=Inherit: Same as input  ParamDataTypeStr=Inherit: Same as input
  R_choke7 : Gain  Commented=on  Gain=-acom  SaturateOnIntegerOverflow=on  OutDataTypeStr=Inherit: Same as input  ParamDataTypeStr=Inherit: Same as input
  R_choke8 : Gain  Commented=on  Gain=bcom  SaturateOnIntegerOverflow=on  OutDataTypeStr=Inherit: Same as input  ParamDataTypeStr=Inherit: Same as input
  R_choke9 : Gain  Commented=on  Gain=lam  SaturateOnIntegerOverflow=on  OutDataTypeStr=Inherit: Same as input  ParamDataTypeStr=Inherit: Same as input
  Scope{,3..7,10..13} (10 alike) : Scope
      Scope settings: ActiveDisplayYMinimum=-0.0194  ActiveDisplayYMaximum=0.04689
      Scope10 settings: ActiveDisplayYMinimum=-0.00511  ActiveDisplayYMaximum=0.046
      Scope11 settings: ActiveDisplayYMinimum=-0.1125  ActiveDisplayYMaximum=0.0125  DataLoggingVariableName=ScopeData2
      Scope12 settings: ActiveDisplayYMinimum=0.46883  ActiveDisplayYMaximum=1.25548  DataLoggingVariableName=ScopeData3
      Scope13 settings: ActiveDisplayYMinimum=-0.00656  ActiveDisplayYMaximum=0.05904  DataLoggingVariableName=ScopeData4
      Scope3 settings: ActiveDisplayYMinimum=-0.12696  ActiveDisplayYMaximum=1.14248
      Scope4 settings: ActiveDisplayYMinimum=-2.8E-5  ActiveDisplayYMaximum=2.4E-5  DataLoggingVariableName=ScopeData5
      Scope5 settings: ActiveDisplayYMinimum=-0.00823  ActiveDisplayYMaximum=0.07404  DataLoggingVariableName=ScopeData7
      Scope6 settings: ActiveDisplayYMinimum=-4.9E-5  ActiveDisplayYMaximum=-0  DataLoggingVariableName=ScopeData4
      Scope7 settings: ActiveDisplayYMinimum=0.9  ActiveDisplayYMaximum=1.1  DataLoggingVariableName=ScopeData14
  Selector : Selector  InputPortWidth=2  IndexOptions=Index vector (dialog)  Indices=[2 1]  OutputSizes=1
  Sum : Sum  Inputs=+--+  SaturateOnIntegerOverflow=on
  Sum1 : Sum  Inputs=|++  SaturateOnIntegerOverflow=on
  Sum13 : Sum  Commented=on  Inputs=+++  SaturateOnIntegerOverflow=on
  Sum{3,5,14,16,19,21,23,25} (8 alike) : Sum  Commented=on  Inputs=|+-  SaturateOnIntegerOverflow=on
  Sum{4,15,20,24} (4 alike) : Sum  Commented=on  Inputs=|++  SaturateOnIntegerOverflow=on
  Sum17 : Sum  Commented=on  Inputs=-+  SaturateOnIntegerOverflow=on
  Sum18 : Sum  Commented=on  Inputs=+++  SaturateOnIntegerOverflow=on
  Sum22 : Sum  Commented=on  Inputs=-+  SaturateOnIntegerOverflow=on
  Sum26 : Sum  Inputs=|+-  SaturateOnIntegerOverflow=on
  Sum6 : Sum  Inputs=|++  SaturateOnIntegerOverflow=on
  Sum9 : Sum  Inputs=-+-  SaturateOnIntegerOverflow=on
  Switch2 : Switch  Criteria=u2 ~= 0  Threshold=0.5  InputSameDT=off
  Switch3 : Switch  Criteria=u2 ~= 0  Threshold=0.5  InputSameDT=off
  Terminator : Terminator
  Transport Delay{6..7,10..11} (4 alike) : TransportDelay  Commented=on  DelayTime=DataDelay(4,1)
  Transport Delay{4..5,8..9} (4 alike) : TransportDelay  Commented=on  DelayTime=DataDelay(2,2)
  output : Subsystem
  w0 : Constant
  xy->dq : Subsystem
  m : Outport
  isxy : Outport  Port=2
  GBxy : Outport  Port=3
  tag scope: DWES3DT=global, Dess3=global, Hess3=global, WreES3=global
  wires:
  Selector/1 -> R_choke1/1
  Sum/1 -> Scope4/1, R_choke3/1
  R_choke3/1 -> Switch2/3
  Ground/1 -> Bistable2/2
  R_choke2/1 -> Sum/4
  R_choke/1 -> Sum/3
  [ucxy] -> Sum/2
  output/1(m) -> m/1
  NOT/1 -> " control1"/Enable
  R_choke1/1 -> R_choke2/1
  Bistable2/1 -> NOT/1, [outage]
  Isxy/1 -> Switch3/3
  [isxy] -> xy->dq/1(Ixy)
  [isxy] -> output/1(is_xy)
  output/2(isxy) -> isxy/1
  [xy_dq_delta] -> " control1"/3(delta)
  xy->dq/1(Idq) -> [isdq], Scope/1
  Bistable2/2 -> Terminator/1
  outage/1 -> Bistable2/1
  [outage] -> Switch2/2, Switch3/2
  [isdq] -> " control1"/2(isdq)
  " control1"/1(ucx) -> Mux/1
  Switch2/1 -> Isxy/1
  Switch3/1 -> R_choke/1, Selector/1, [isxy]
  Mux/1 -> Scope12/1, [ucxy]
  [usdq] -> " control1"/1(usdq)
  output/3(GBxy) -> GBxy/1
  Constant1/1 -> Switch2/1, Switch3/1
  " control1"/2(ucy) -> Mux/2
  [usdq] -> Product2/1
  Add1/1 -> output/2(Pe), Scope5/1  "Pess1"
  Product2/1 -> Add1/1
  [isdq] -> Product2/2
  Product1/1 -> Scope6/1, [DWES3DT], Int2/1
  Int2/1 -> Sum26/1
  w0/1 -> Sum26/2
  Sum9/1 -> Product1/1, Scope11/1
  Constant/1 -> Divide/1
  Divide/1 -> Product1/2, Scope7/1
  [Hess3] -> Divide/2
  us_xy/1 -> Mux4/1, Sum/1
  Fcn3/1 -> Mux3/1
  Fcn4/1 -> Mux3/2
  Mux4/1 -> Fcn3/1, Fcn4/1
  [xy_dq_delta] -> Mux4/2, xy->dq/2(Theta)
  Mux3/1 -> Scope3/1, [usdq]
  Gain4/1 -> Sum9/3
  Constant4/1 -> Sum9/2
  Product4/1 -> Sum9/1
  Int1/1 -> [xy_dq_delta]
  Add2/1 -> Gain4/1, Scope10/1  "Pess1"
  [usdq] -> Product3/1
  [isdq] -> Product3/2
  Product3/1 -> Add2/1
  [Dess3] -> Product4/1
  Gain1/1 -> Int1/1
  R_choke8/1 -> Sum13/2
  Transport Delay9/1 -> Goto23/1
  Sum6/1 -> [Hess3]  "Hess3"
  From42/1 -> Sum21/1
  R_choke4/1 -> Integrator3/1
  From39/1 -> Sum23/2
  From9/1 -> Sum3/1
  From40/1 -> Sum25/2
  From24/1 -> Sum5/1
  From27/1 -> Sum5/2
  Transport Delay4/1 -> Goto20/1
  From45/1 -> Sum23/1
  Constant2/1 -> Sum6/1
  Sum1/1 -> [Dess3]  "Dess3"
  Constant3/1 -> Sum1/1
  From28/1 -> Sum14/1
  Sum20/1 -> R_choke12/1
  From26/1 -> Sum3/2
  From30/1 -> Sum14/2
  From29/1 -> Sum16/1
  R_choke13/1 -> Sum18/3
  Sum24/1 -> R_choke11/1, R_choke10/1
  R_choke7/1 -> Sum13/1
  R_choke9/1 -> Sum13/3
  From44/1 -> Sum21/2
  Sum4/1 -> R_choke7/1, R_choke4/1
  R_choke11/1 -> Sum18/1
  Transport Delay5/1 -> Goto22/1
  Integrator5/1 -> Goto25/1
  Transport Delay10/1 -> Goto17/1
  From38/1 -> Sum25/1
  Integrator6/1 -> Goto24/1, Sum22/1
  Transport Delay7/1 -> Goto19/1
  R_choke10/1 -> Integrator5/1
  Integrator3/1 -> Goto18/1
  Transport Delay6/1 -> Goto21/1
  Transport Delay11/1 -> Goto14/1
  Transport Delay8/1 -> Goto15/1
  Sum17/1 -> R_choke9/1
  From31/1 -> Sum16/2
  Sum22/1 -> R_choke13/1
  Sum15/1 -> R_choke8/1
  From43/1 -> Sum19/2
  R_choke12/1 -> Sum18/2
  Sum18/1 -> Integrator6/1
  [deltaDess3] -> Gain/1, Sum1/2
  Integrator4/1 -> Goto16/1, Sum17/1
  Sum13/1 -> Integrator4/1
  From41/1 -> Sum19/1
  Sum26/1 -> [WreES3], Gain1/1, Scope13/1, Product4/2
  Gain/1 -> Sum17/2
  Gain2/1 -> Sum22/2
  From14/1 -> Transport Delay7/1
  From32/1 -> Transport Delay6/1
  From34/1 -> Transport Delay11/1
  From36/1 -> Transport Delay10/1
  From37/1 -> Transport Delay9/1
  From35/1 -> Transport Delay8/1
  From33/1 -> Transport Delay5/1
  From25/1 -> Transport Delay4/1
  [deltaHess3] -> Gain2/1, Sum6/2
  Gain3/1 -> Sum4/1
  Sum3/1 -> Gain3/1
  Sum5/1 -> Gain5/1
  Gain5/1 -> Sum4/2
  Sum14/1 -> Gain6/1
  Gain6/1 -> Sum15/1
  Sum16/1 -> Gain7/1
  Gain7/1 -> Sum15/2
  Sum23/1 -> Gain8/1
  Gain8/1 -> Sum24/1
  Gain9/1 -> Sum24/2
  Sum25/1 -> Gain9/1
  Sum19/1 -> Gain10/1
  Gain10/1 -> Sum20/1
  Gain11/1 -> Sum20/2
  Sum21/1 -> Gain11/1

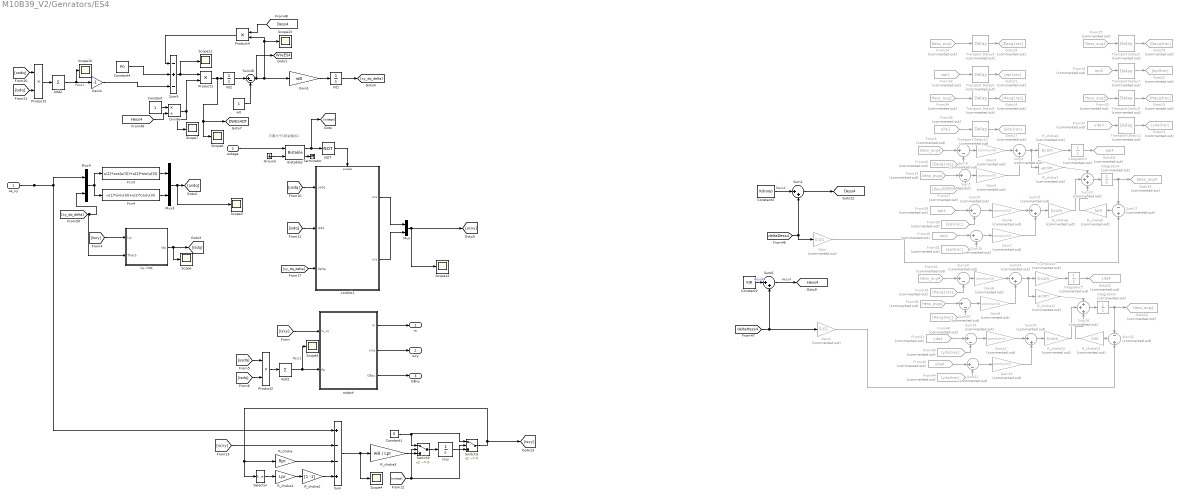
== system M10B39_V2/Genrators/ES4 ==
  note: 只要大于0就会输出1
  us_xy : Inport
  outage : Inport  Port=2
  " control1" : Subsystem
  Add1 : Sum  Inputs=+
  Add2 : Sum  Inputs=+
  Bistable2 : powerlib_meascontrol/Logic/Bistable  Qpriority=Set  ic=0  Ts=0
  Constant : Constant
  Constant1 : Constant  Value=0
  Constant2 : Constant  Value=KIR
  Constant3 : Constant  Value=Kdroop
  Constant4 : Constant  Value=P0
  Divide : Product  Inputs=*/
  Fcn3 : Fcn  Expr=u(1)*cos(u(3))+u(2)*sin(u(3))
  Fcn4 : Fcn  Expr=-u(1)*sin(u(3))+u(2)*cos(u(3))
  From14 : From  Commented=on  GotoTag=Dess_avg1  TagVisibility=global
  From24 : From  Commented=on  GotoTag=Dess_avg4  TagVisibility=global
  From25 : From  Commented=on  GotoTag=Dess_avg3  TagVisibility=global
  From26 : From  Commented=on  GotoTag=Davg1rec
  From27 : From  Commented=on  GotoTag=Davg3rec
  From28 : From  Commented=on  GotoTag=epi4  TagVisibility=global
  From29 : From  Commented=on  GotoTag=epi4  TagVisibility=global
  From30 : From  Commented=on  GotoTag=epi1rec
  From31 : From  Commented=on  GotoTag=epi3rec
  From32 : From  Commented=on  GotoTag=epi1  TagVisibility=global
  From33 : From  Commented=on  GotoTag=epi3  TagVisibility=global
  From34 : From  Commented=on  GotoTag=Hess_avg1  TagVisibility=global
  From35 : From  Commented=on  GotoTag=Hess_avg3  TagVisibility=global
  From36 : From  Commented=on  GotoTag=yita1  TagVisibility=global
  From37 : From  Commented=on  GotoTag=yita3  TagVisibility=global
  From38 : From  Commented=on  GotoTag=Hess_avg4  TagVisibility=global
  From39 : From  Commented=on  GotoTag=Havg1rec
  From40 : From  Commented=on  GotoTag=Havg3rec
  From41 : From  Commented=on  GotoTag=yita4  TagVisibility=global
  From42 : From  Commented=on  GotoTag=yita4  TagVisibility=global
  From43 : From  Commented=on  GotoTag=yita1rec
  From44 : From  Commented=on  GotoTag=yita3rec
  From45 : From  Commented=on  GotoTag=Hess_avg4  TagVisibility=global
  From9 : From  Commented=on  GotoTag=Dess_avg4  TagVisibility=global
  Gain : Gain  Commented=on  Gain=0.01
  Gain1 : Gain  Gain=wB  SaturateOnIntegerOverflow=on  OutDataTypeStr=Inherit: Same as input  ParamDataTypeStr=Inherit: Same as input
  Gain{3,6,8,12} (4 alike) : Gain  Commented=on  Gain=commun(4)
  Gain{5,7,9,13} (4 alike) : Gain  Commented=on  Gain=commun(3)
  Gain2 : Gain  Commented=on  Gain=0.01
  Gain4 : Gain  Gain=-1
  Goto14 : Goto  Commented=on  GotoTag=Havg1rec
  Goto15 : Goto  Commented=on  GotoTag=Havg3rec
  Goto16 : Goto  Commented=on  GotoTag=Dess_avg4  TagVisibility=global
  Goto17 : Goto  Commented=on  GotoTag=yita1rec
  Goto18 : Goto  Commented=on  GotoTag=epi4  TagVisibility=global
  Goto19 : Goto  Commented=on  GotoTag=Davg1rec
  Goto20 : Goto  Commented=on  GotoTag=Davg3rec
  Goto21 : Goto  Commented=on  GotoTag=epi1rec
  Goto22 : Goto  Commented=on  GotoTag=epi3rec
  Goto23 : Goto  Commented=on  GotoTag=yita3rec
  Goto24 : Goto  Commented=on  GotoTag=Hess_avg4  TagVisibility=global
  Goto25 : Goto  Commented=on  GotoTag=yita4  TagVisibility=global
  Ground : Ground
  Int1 : Integrator  InitialCondition=Dels_hvdc
  Int2 : Integrator  InitialCondition=1
  Integrator{3..6} (4 alike) : Integrator  Commented=on
  Isxy : Integrator  InitialCondition=[Is_xA_0 Is_yA_0]
  Mux : Mux  Inputs=2
  Mux3 : Mux  Inputs=2
  Mux4 : Mux  Inputs=2
  NOT : Logic  Operator=NOT  AllPortsSameDT=off  OutDataTypeStr=boolean
  Product1 : Product
  Product2 : Product  RndMeth=Zero
  Product3 : Product  RndMeth=Zero
  Product4 : Product
  R_choke : Gain  Gain=Rpr  SaturateOnIntegerOverflow=on  OutDataTypeStr=Inherit: Same as input  ParamDataTypeStr=Inherit: Same as input
  R_choke1 : Gain  Gain=Lpr  SaturateOnIntegerOverflow=on  OutDataTypeStr=Inherit: Same as input  ParamDataTypeStr=Inherit: Same as input
  R_choke10 : Gain  Commented=on  Gain=-bcom  SaturateOnIntegerOverflow=on  OutDataTypeStr=Inherit: Same as input  ParamDataTypeStr=Inherit: Same as input
  R_choke11 : Gain  Commented=on  Gain=-acom  SaturateOnIntegerOverflow=on  OutDataTypeStr=Inherit: Same as input  ParamDataTypeStr=Inherit: Same as input
  R_choke12 : Gain  Commented=on  Gain=bcom  SaturateOnIntegerOverflow=on  OutDataTypeStr=Inherit: Same as input  ParamDataTypeStr=Inherit: Same as input
  R_choke13 : Gain  Commented=on  Gain=lam  SaturateOnIntegerOverflow=on  OutDataTypeStr=Inherit: Same as input  ParamDataTypeStr=Inherit: Same as input
  R_choke2 : Gain  Gain=[1 -1]  SaturateOnIntegerOverflow=on  OutDataTypeStr=Inherit: Same as input  ParamDataTypeStr=Inherit: Same as input
  R_choke3 : Gain  Gain=wB / Lpr  SaturateOnIntegerOverflow=on  OutDataTypeStr=Inherit: Same as input  ParamDataTypeStr=Inherit: Same as input
  R_choke4 : Gain  Commented=on  Gain=-bcom  SaturateOnIntegerOverflow=on  OutDataTypeStr=Inherit: Same as input  ParamDataTypeStr=Inherit: Same as input
  R_choke7 : Gain  Commented=on  Gain=-acom  SaturateOnIntegerOverflow=on  OutDataTypeStr=Inherit: Same as input  ParamDataTypeStr=Inherit: Same as input
  R_choke8 : Gain  Commented=on  Gain=bcom  SaturateOnIntegerOverflow=on  OutDataTypeStr=Inherit: Same as input  ParamDataTypeStr=Inherit: Same as input
  R_choke9 : Gain  Commented=on  Gain=lam  SaturateOnIntegerOverflow=on  OutDataTypeStr=Inherit: Same as input  ParamDataTypeStr=Inherit: Same as input
  Scope{,3..7,10..13} (10 alike) : Scope
      Scope settings: ActiveDisplayYMinimum=-0.0194  ActiveDisplayYMaximum=0.04689
      Scope10 settings: ActiveDisplayYMinimum=-6.46308  ActiveDisplayYMaximum=-6.45084
      Scope11 settings: ActiveDisplayYMinimum=-0.1125  ActiveDisplayYMaximum=0.0125  DataLoggingVariableName=ScopeData2
      Scope12 settings: ActiveDisplayYMinimum=0.46883  ActiveDisplayYMaximum=1.25548  DataLoggingVariableName=ScopeData3
      Scope13 settings: ActiveDisplayYMinimum=-0.00656  ActiveDisplayYMaximum=0.05904  DataLoggingVariableName=ScopeData4
      Scope3 settings: ActiveDisplayYMinimum=-0.12696  ActiveDisplayYMaximum=1.14248
      Scope4 settings: ActiveDisplayYMinimum=-2.8E-5  ActiveDisplayYMaximum=2.4E-5  DataLoggingVariableName=ScopeData5
      Scope5 settings: ActiveDisplayYMinimum=-0.00823  ActiveDisplayYMaximum=0.07404  DataLoggingVariableName=ScopeData7
      Scope6 settings: ActiveDisplayYMinimum=-4.9E-5  ActiveDisplayYMaximum=-0  DataLoggingVariableName=ScopeData4
      Scope7 settings: ActiveDisplayYMinimum=0.9  ActiveDisplayYMaximum=1.1  DataLoggingVariableName=ScopeData14
  Selector : Selector  InputPortWidth=2  IndexOptions=Index vector (dialog)  Indices=[2 1]  OutputSizes=1
  Sum : Sum  Inputs=+--+  SaturateOnIntegerOverflow=on
  Sum1 : Sum  Inputs=|++  SaturateOnIntegerOverflow=on
  Sum13 : Sum  Commented=on  Inputs=+++  SaturateOnIntegerOverflow=on
  Sum{3,5,14,16,19,21,23,25} (8 alike) : Sum  Commented=on  Inputs=|+-  SaturateOnIntegerOverflow=on
  Sum{4,15,20,24} (4 alike) : Sum  Commented=on  Inputs=|++  SaturateOnIntegerOverflow=on
  Sum17 : Sum  Commented=on  Inputs=-+  SaturateOnIntegerOverflow=on
  Sum18 : Sum  Commented=on  Inputs=+++  SaturateOnIntegerOverflow=on
  Sum22 : Sum  Commented=on  Inputs=-+  SaturateOnIntegerOverflow=on
  Sum26 : Sum  Inputs=|+-  SaturateOnIntegerOverflow=on
  Sum6 : Sum  Inputs=|++  SaturateOnIntegerOverflow=on
  Sum9 : Sum  Inputs=-+-  SaturateOnIntegerOverflow=on
  Switch2 : Switch  Criteria=u2 ~= 0  Threshold=0.5  InputSameDT=off
  Switch3 : Switch  Criteria=u2 ~= 0  Threshold=0.5  InputSameDT=off
  Terminator : Terminator
  Transport Delay{4,6,8,10} (4 alike) : TransportDelay  Commented=on  DelayTime=DataDelay(1,1)
  Transport Delay{5,7,9,11} (4 alike) : TransportDelay  Commented=on  DelayTime=DataDelay(3,2)
  output : Subsystem
  w0 : Constant
  xy->dq : Subsystem
  m : Outport
  isxy : Outport  Port=2
  GBxy : Outport  Port=3
  tag scope: DWES4DT=global, Dess4=global, Hess4=global, WreES4=global
  wires:
  Selector/1 -> R_choke1/1
  Sum/1 -> Scope4/1, R_choke3/1
  R_choke3/1 -> Switch2/3
  Ground/1 -> Bistable2/2
  R_choke2/1 -> Sum/4
  R_choke/1 -> Sum/3
  [ucxy] -> Sum/2
  output/1(m) -> m/1
  NOT/1 -> " control1"/Enable
  R_choke1/1 -> R_choke2/1
  Bistable2/1 -> NOT/1, [outage]
  Isxy/1 -> Switch3/3
  [isxy] -> xy->dq/1(Ixy)
  [isxy] -> output/1(is_xy)
  output/2(isxy) -> isxy/1
  [xy_dq_delta] -> " control1"/3(delta)
  xy->dq/1(Idq) -> [isdq], Scope/1
  Bistable2/2 -> Terminator/1
  outage/1 -> Bistable2/1
  [outage] -> Switch2/2, Switch3/2
  [isdq] -> " control1"/2(isdq)
  " control1"/1(ucx) -> Mux/1
  Switch2/1 -> Isxy/1
  Switch3/1 -> R_choke/1, Selector/1, [isxy]
  Mux/1 -> Scope12/1, [ucxy]
  [usdq] -> " control1"/1(usdq)
  output/3(GBxy) -> GBxy/1
  Constant1/1 -> Switch2/1, Switch3/1
  " control1"/2(ucy) -> Mux/2
  [usdq] -> Product2/1
  Add1/1 -> output/2(Pe), Scope5/1  "Pess1"
  Product2/1 -> Add1/1
  [isdq] -> Product2/2
  Product1/1 -> Scope6/1, [DWES4DT], Int2/1
  Sum26/1 -> [WreES4], Gain1/1, Scope13/1, Product4/2
  Int2/1 -> Sum26/1
  w0/1 -> Sum26/2
  Sum9/1 -> Product1/1, Scope11/1
  Constant/1 -> Divide/1
  Divide/1 -> Product1/2, Scope7/1
  [Hess4] -> Divide/2
  us_xy/1 -> Mux4/1, Sum/1
  Fcn3/1 -> Mux3/1
  Fcn4/1 -> Mux3/2
  Mux4/1 -> Fcn3/1, Fcn4/1
  [xy_dq_delta] -> Mux4/2, xy->dq/2(Theta)
  Mux3/1 -> Scope3/1, [usdq]
  Gain4/1 -> Sum9/3
  Constant4/1 -> Sum9/2
  Product4/1 -> Sum9/1
  Int1/1 -> [xy_dq_delta]
  Add2/1 -> Gain4/1, Scope10/1  "Pess1"
  [usdq] -> Product3/1
  [isdq] -> Product3/2
  Product3/1 -> Add2/1
  [Dess4] -> Product4/1
  Gain1/1 -> Int1/1
  Integrator4/1 -> Sum17/1, Goto16/1
  From30/1 -> Sum14/2
  From31/1 -> Sum16/2
  [deltaDess4] -> Sum1/2, Gain/1
  R_choke9/1 -> Sum13/3
  Sum20/1 -> R_choke12/1
  Constant2/1 -> Sum6/1  "Hess4"
  From29/1 -> Sum16/1
  Constant3/1 -> Sum1/1  "Dess4"
  Sum24/1 -> R_choke11/1, R_choke10/1
  Integrator3/1 -> Goto18/1
  Sum15/1 -> R_choke8/1
  From26/1 -> Sum3/2
  Transport Delay4/1 -> Goto19/1
  Transport Delay5/1 -> Goto20/1
  R_choke4/1 -> Integrator3/1
  Transport Delay7/1 -> Goto22/1
  From39/1 -> Sum23/2
  Transport Delay8/1 -> Goto14/1
  Sum17/1 -> R_choke9/1
  Transport Delay6/1 -> Goto21/1
  Sum13/1 -> Integrator4/1
  Transport Delay10/1 -> Goto17/1
  From40/1 -> Sum25/2
  Transport Delay9/1 -> Goto15/1
  Transport Delay11/1 -> Goto23/1
  From45/1 -> Sum23/1
  R_choke10/1 -> Integrator5/1
  From42/1 -> Sum21/1
  R_choke8/1 -> Sum13/2
  From28/1 -> Sum14/1
  From24/1 -> Sum5/1
  R_choke7/1 -> Sum13/1
  Sum18/1 -> Integrator6/1
  R_choke12/1 -> Sum18/2
  From38/1 -> Sum25/1
  Sum22/1 -> R_choke13/1
  R_choke13/1 -> Sum18/3
  From41/1 -> Sum19/1
  Sum4/1 -> R_choke7/1, R_choke4/1
  From44/1 -> Sum21/2
  R_choke11/1 -> Sum18/1
  From27/1 -> Sum5/2
  From9/1 -> Sum3/1
  Integrator6/1 -> Sum22/1, Goto24/1
  From43/1 -> Sum19/2
  Integrator5/1 -> Goto25/1
  [deltaHess4] -> Gain2/1, Sum6/2
  Gain/1 -> Sum17/2
  Gain2/1 -> Sum22/2
  From14/1 -> Transport Delay4/1
  From32/1 -> Transport Delay6/1
  From34/1 -> Transport Delay8/1
  From36/1 -> Transport Delay10/1
  From25/1 -> Transport Delay5/1
  From33/1 -> Transport Delay7/1
  From35/1 -> Transport Delay9/1
  From37/1 -> Transport Delay11/1
  Sum3/1 -> Gain3/1
  Gain3/1 -> Sum4/1
  Sum5/1 -> Gain5/1
  Gain5/1 -> Sum4/2
  Gain6/1 -> Sum15/1
  Sum14/1 -> Gain6/1
  Sum16/1 -> Gain7/1
  Gain7/1 -> Sum15/2
  Sum23/1 -> Gain8/1
  Gain8/1 -> Sum24/1
  Gain9/1 -> Sum24/2
  Sum25/1 -> Gain9/1
  Gain12/1 -> Sum20/1
  Sum19/1 -> Gain12/1
  Sum21/1 -> Gain13/1
  Gain13/1 -> Sum20/2
  Sum1/1 -> [Dess4]
  Sum6/1 -> [Hess4]  "Hess4"
